simulink model "analogicalgates"  (R2015a)
settings: Solver=ode45  StartTime=0.0  StopTime=10.0  RelTol=1e-3
settings Model: Creator=Elena  LastModifiedBy=Elena

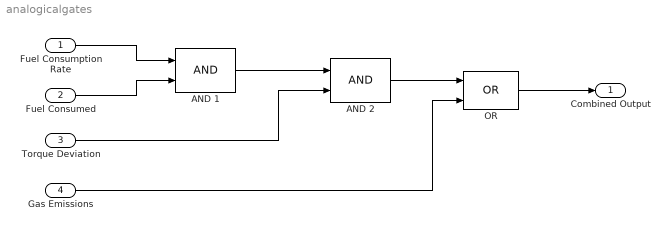
== system analogicalgates ==
  Fuel Consumption Rate : Inport
  Fuel Consumed : Inport  Port=2
  Torque Deviation : Inport  Port=3
  Gas Emissions : Inport  Port=4
  AND 1 : Logic  IconShape=distinctive  AllPortsSameDT=off  OutDataTypeStr=boolean
  AND 2 : Logic  IconShape=distinctive  AllPortsSameDT=off  OutDataTypeStr=boolean
  OR : Logic  Operator=OR  IconShape=distinctive  AllPortsSameDT=off  OutDataTypeStr=boolean
  Combined Output : Outport
  wires:
  Fuel Consumption Rate/1 -> AND 1/1
  Fuel Consumed/1 -> AND 1/2
  Torque Deviation/1 -> AND 2/2
  AND 1/1 -> AND 2/1
  AND 2/1 -> OR/1
  Gas Emissions/1 -> OR/2
  OR/1 -> Combined Output/1
